simulink model "Single_Cell_BMS"  (R2024a)
settings: Solver=VariableStepAuto  StartTime=0.0  StopTime=1180  RelTol=1e-3
undefined symbols (not defined in the file): C1_LUT, Capacity_LUT, Cell_area, Cell_cp, Cell_mass, DiscIntNeverNeededParam, Em_LUT, H_con, R1_LUT, Ro_LUT, SOC_LUT, T_init, Temp_LUT
settings Model: Creator=gopin  LastModifiedBy=gopin

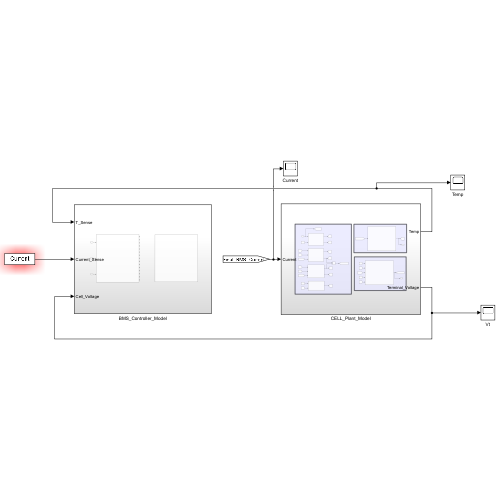
[thumbnail: Simulink's stored preview of the top-level diagram]
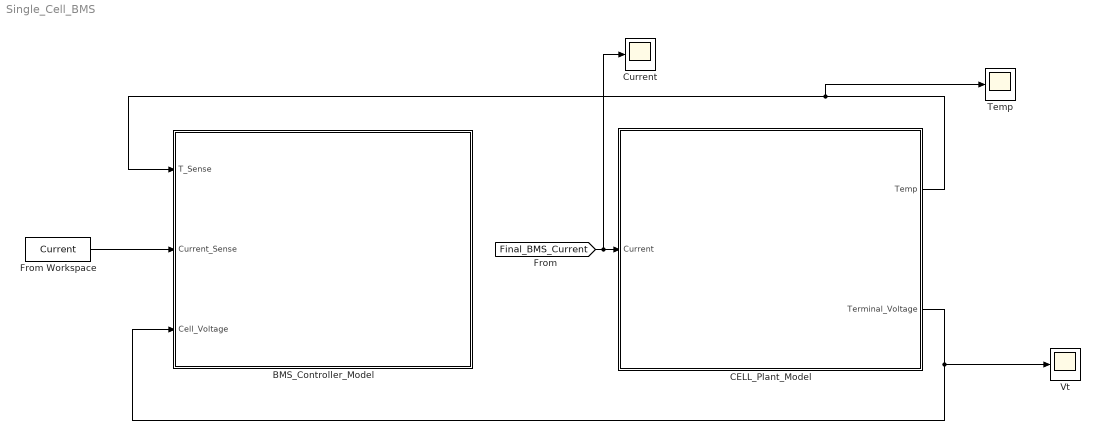
== system Single_Cell_BMS ==
  BMS_Controller_Model : Subsystem
  CELL_Plant_Model : Subsystem
  Current : Scope
  From Workspace : FromWorkspace  VariableName=Current
  Temp : Scope
  Vt : Scope
  wires:
  [Final_BMS_Current] -> Current/1, CELL_Plant_Model/1(Current)
  CELL_Plant_Model/2(Terminal_Voltage) -> BMS_Controller_Model/3(Cell_Voltage), Vt/1
  CELL_Plant_Model/1(Temp) -> Temp/1, BMS_Controller_Model/1(T_Sense)
  From Workspace/1 -> BMS_Controller_Model/2(Current_Sense)

== system Single_Cell_BMS/BMS_Controller_Model ==
  T_Sense : Inport
  Current_Sense : Inport  Port=2
  Cell_Voltage : Inport  Port=3
  Protection_Logc : Subsystem
  SOC_Estimation : Subsystem
  wires:
  Cell_Voltage/1 -> Protection_Logc/1(Cell_voltage)
  Current_Sense/1 -> Protection_Logc/2(C-Sense)
  T_Sense/1 -> Protection_Logc/3(T_Sense)

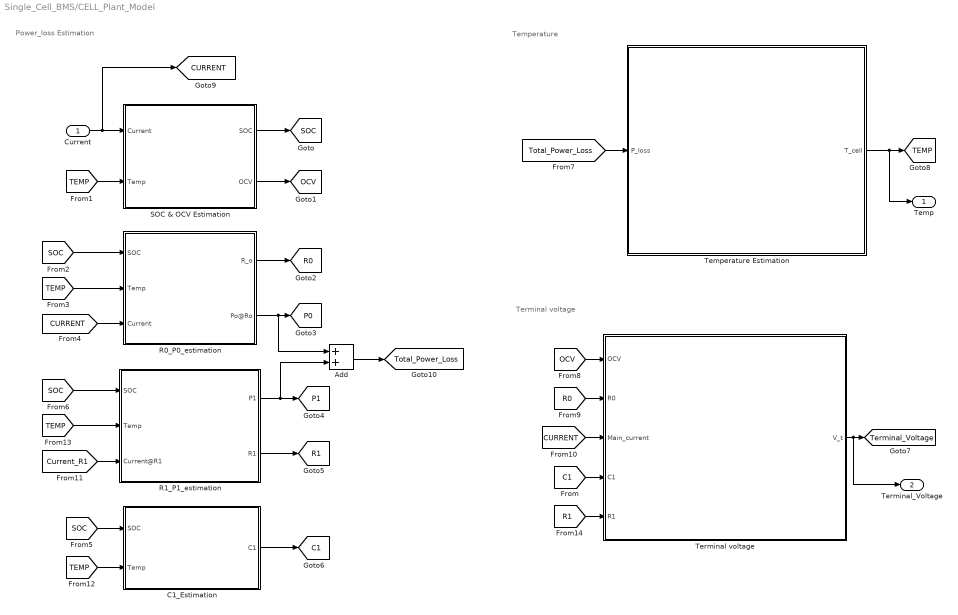
== system Single_Cell_BMS/CELL_Plant_Model ==
  note: Power_loss Estimation
  note: Temperature
  note: Terminal voltage
  Current : Inport
  Add : Sum
  C1_Estimation : Subsystem
  "R0_P0_estimation " : Subsystem
  R1_P1_estimation : Subsystem
  SOC & OCV Estimation : Subsystem
  Temperature Estimation : Subsystem
  Terminal voltage : Subsystem
  Temp : Outport
  Terminal_Voltage : Outport  Port=2
  tag scope: C1=global, CURRENT=global, OCV=global, P0=global, P1=global, R0=global, R1=global, SOC=global, TEMP=global, Terminal_Voltage=global, Total_Power_Loss=global
  wires:
  Current/1 -> [CURRENT], SOC & OCV Estimation/1(Current)
  [TEMP] -> SOC & OCV Estimation/2(Temp)
  [SOC] -> "R0_P0_estimation "/1(SOC)
  [TEMP] -> "R0_P0_estimation "/2(Temp)
  [CURRENT] -> "R0_P0_estimation "/3(Current)
  [SOC] -> R1_P1_estimation/1(SOC)
  [TEMP] -> R1_P1_estimation/2(Temp)
  [Current_R1] -> R1_P1_estimation/3(Current@R1)
  [SOC] -> C1_Estimation/1(SOC)
  [TEMP] -> C1_Estimation/2(Temp)
  [Total_Power_Loss] -> Temperature Estimation/1(P_loss)
  [OCV] -> Terminal voltage/1(OCV)
  [R0] -> Terminal voltage/2(R0)
  [CURRENT] -> Terminal voltage/3(Main_current)
  [C1] -> Terminal voltage/4(C1)
  [R1] -> Terminal voltage/5(R1)
  SOC & OCV Estimation/1(SOC) -> [SOC]
  SOC & OCV Estimation/2(OCV) -> [OCV]
  "R0_P0_estimation "/1(R_o) -> [R0]
  "R0_P0_estimation "/2(Po@Ro) -> Add/1, [P0]
  R1_P1_estimation/1(P1) -> Add/2, [P1]
  R1_P1_estimation/2(R1) -> [R1]
  C1_Estimation/1(C1) -> [C1]
  Temperature Estimation/1(T_cell) -> Temp/1, [TEMP]
  Terminal voltage/1(V_t) -> Terminal_Voltage/1, [Terminal_Voltage]
  Add/1 -> [Total_Power_Loss]

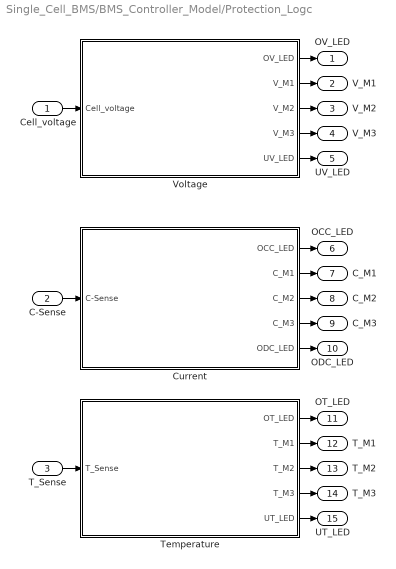
== system Single_Cell_BMS/BMS_Controller_Model/Protection_Logc ==
  Cell_voltage : Inport
  C-Sense : Inport  Port=2
  T_Sense : Inport  Port=3
  Current : Subsystem
  Temperature : Subsystem
  Voltage : Subsystem
  OV_LED : Outport
  V_M1 : Outport  Port=2
  V_M2 : Outport  Port=3
  V_M3 : Outport  Port=4
  UV_LED : Outport  Port=5
  OCC_LED : Outport  Port=6
  C_M1 : Outport  Port=7
  C_M2 : Outport  Port=8
  C_M3 : Outport  Port=9
  ODC_LED : Outport  Port=10
  OT_LED : Outport  Port=11
  T_M1 : Outport  Port=12
  T_M2 : Outport  Port=13
  T_M3 : Outport  Port=14
  UT_LED : Outport  Port=15
  wires:
  Voltage/4(V_M3) -> V_M3/1
  Voltage/1(OV_LED) -> OV_LED/1
  T_Sense/1 -> Temperature/1(T_Sense)
  Voltage/2(V_M1) -> V_M1/1
  Voltage/5(UV_LED) -> UV_LED/1
  Cell_voltage/1 -> Voltage/1(Cell_voltage)
  C-Sense/1 -> Current/1(C-Sense)
  Current/3(C_M2) -> C_M2/1
  Voltage/3(V_M2) -> V_M2/1
  Current/5(ODC_LED) -> ODC_LED/1
  Current/2(C_M1) -> C_M1/1
  Current/4(C_M3) -> C_M3/1
  Temperature/1(OT_LED) -> OT_LED/1
  Temperature/2(T_M1) -> T_M1/1
  Current/1(OCC_LED) -> OCC_LED/1
  Temperature/4(T_M3) -> T_M3/1
  Temperature/3(T_M2) -> T_M2/1
  Temperature/5(UT_LED) -> UT_LED/1

== system Single_Cell_BMS/BMS_Controller_Model/SOC_Estimation ==
  Coloumb Counting Based SOC Estimation : Subsystem
  Voltage Based SOC Estimation : Subsystem

== system Single_Cell_BMS/CELL_Plant_Model/C1_Estimation ==
  SOC : Inport
  Temp : Inport  Port=2
  2-D Lookup Table : Lookup_n-D  BreakpointsForDimension1=SOC_LUT  BreakpointsForDimension2=Temp_LUT  Table=C1_LUT  InternalRulePriority=Speed  RndMeth=Simplest
      settings: InputPortMap=u0,u1
  C1 : Outport
  wires:
  SOC/1 -> 2-D Lookup Table/1
  Temp/1 -> 2-D Lookup Table/2
  2-D Lookup Table/1 -> C1/1

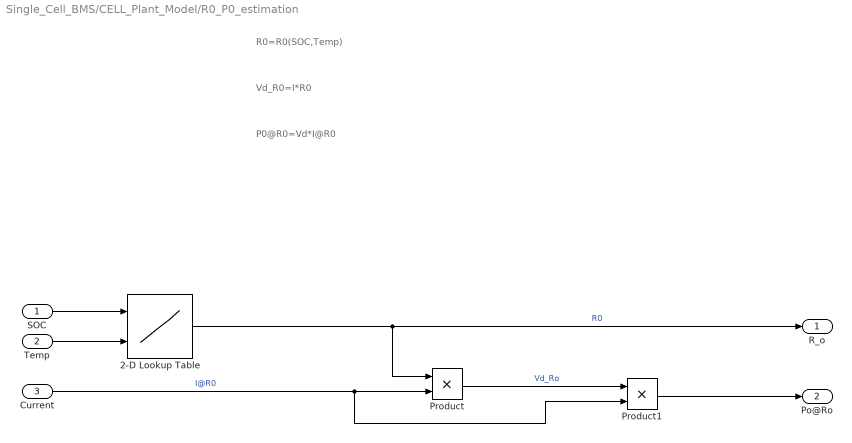
== system Single_Cell_BMS/CELL_Plant_Model/R0_P0_estimation  ==
  note: P0@R0=Vd*I@R0
  note: Vd_R0=I*R0
  note: R0=R0(SOC,Temp)
  SOC : Inport
  Temp : Inport  Port=2
  Current : Inport  Port=3
  2-D Lookup Table : Lookup_n-D  BreakpointsForDimension1=SOC_LUT  BreakpointsForDimension2=Temp_LUT  Table=Ro_LUT  InternalRulePriority=Speed  RndMeth=Simplest
      settings: InputPortMap=u0,u1
  Product : Product
  Product1 : Product
  R_o : Outport
  Po@Ro : Outport  Port=2
  wires:
  Temp/1 -> 2-D Lookup Table/2
  2-D Lookup Table/1 -> Product/1, R_o/1  "R0"
  Current/1 -> Product1/2, Product/2  "I@R0"
  Product/1 -> Product1/1  "Vd_Ro"
  Product1/1 -> Po@Ro/1
  SOC/1 -> 2-D Lookup Table/1

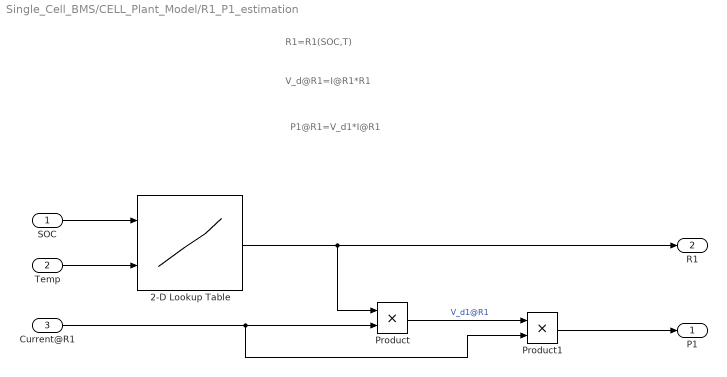
== system Single_Cell_BMS/CELL_Plant_Model/R1_P1_estimation ==
  note: P1@R1=V_d1*I@R1
  note: V_d@R1=I@R1*R1
  note: R1=R1(SOC,T)
  SOC : Inport
  Temp : Inport  Port=2
  Current@R1 : Inport  Port=3
  2-D Lookup Table : Lookup_n-D  BreakpointsForDimension1=SOC_LUT  BreakpointsForDimension2=Temp_LUT  Table=R1_LUT  InternalRulePriority=Speed  RndMeth=Simplest
      settings: InputPortMap=u0,u1
  Product : Product
  Product1 : Product
  P1 : Outport
  R1 : Outport  Port=2
  wires:
  SOC/1 -> 2-D Lookup Table/1
  Temp/1 -> 2-D Lookup Table/2
  2-D Lookup Table/1 -> Product/1, R1/1
  Current@R1/1 -> Product1/2, Product/2
  Product/1 -> Product1/1  "V_d1@R1"
  Product1/1 -> P1/1

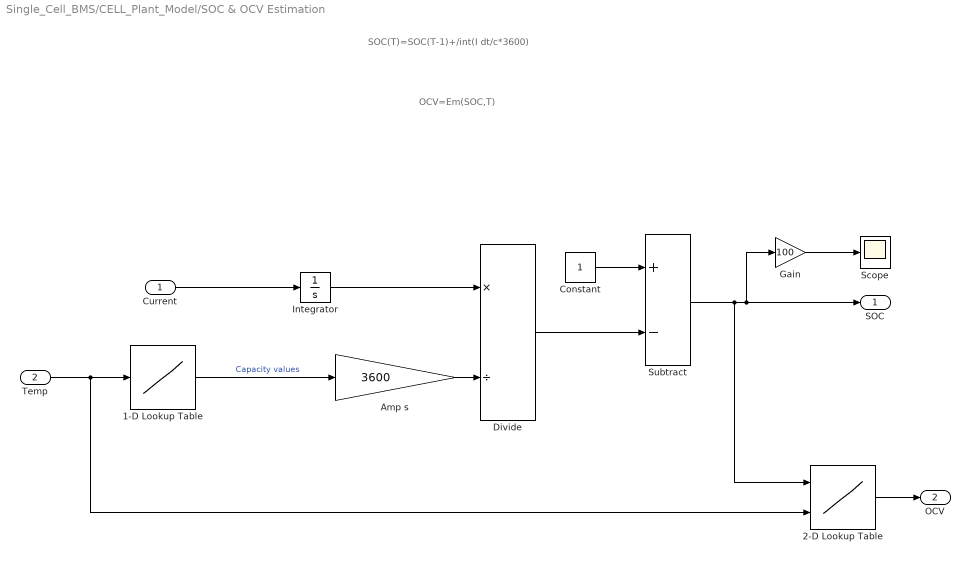
== system Single_Cell_BMS/CELL_Plant_Model/SOC & OCV Estimation ==
  note: SOC(T)=SOC(T-1)+/int(I dt/c*3600)
  note: OCV=Em(SOC,T)
  Current : Inport  OutDataTypeStr=double  PortDimensions=1  SampleTime=0
  Temp : Inport  Port=2  OutDataTypeStr=double  PortDimensions=1  SampleTime=0
  1-D Lookup Table : Lookup_n-D  NumberOfTableDimensions=1  BreakpointsForDimension1=Temp_LUT  Table=Capacity_LUT  InternalRulePriority=Speed  RndMeth=Simplest
  2-D Lookup Table : Lookup_n-D  BreakpointsForDimension1=SOC_LUT  BreakpointsForDimension2=Temp_LUT  Table=Em_LUT  InternalRulePriority=Speed  RndMeth=Simplest
      settings: InputPortMap=u0,u1
  Amp s : Gain  Gain=3600
  Constant : Constant
  Divide : Product  Inputs=*/
  Gain : Gain  Gain=100
  Integrator : Integrator
  Scope : Scope
  Subtract : Sum  Inputs=+-
  SOC : Outport  OutDataTypeStr=double  PortDimensions=1  SampleTime=0
  OCV : Outport  Port=2  OutDataTypeStr=double  PortDimensions=1  SampleTime=0
  wires:
  2-D Lookup Table/1 -> OCV/1
  1-D Lookup Table/1 -> Amp s/1  "Capacity values"
  Subtract/1 -> Gain/1, SOC/1, 2-D Lookup Table/1
  Gain/1 -> Scope/1
  Current/1 -> Integrator/1
  Amp s/1 -> Divide/2
  Temp/1 -> 1-D Lookup Table/1, 2-D Lookup Table/2
  Integrator/1 -> Divide/1
  Divide/1 -> Subtract/2
  Constant/1 -> Subtract/1

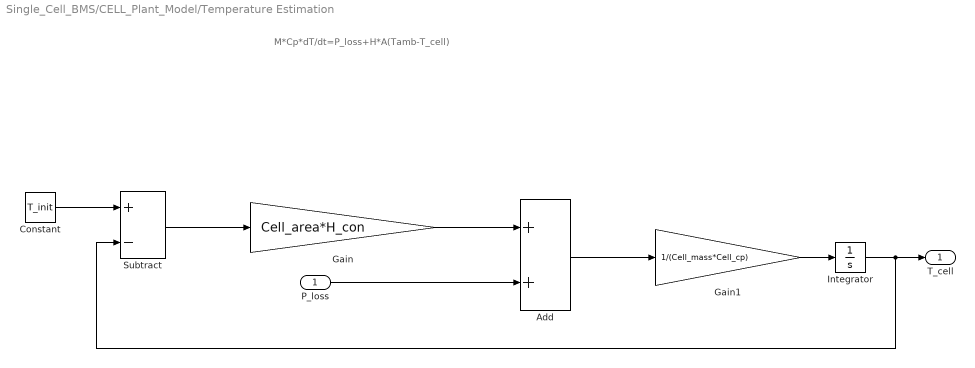
== system Single_Cell_BMS/CELL_Plant_Model/Temperature Estimation ==
  note: M*Cp*dT/dt=P_loss+H*A(Tamb-T_cell)
  P_loss : Inport  OutDataTypeStr=double  PortDimensions=1  SampleTime=0
  Add : Sum
  Constant : Constant  Value=T_init
  Gain : Gain  Gain=Cell_area*H_con
  Gain1 : Gain  Gain=1/(Cell_mass*Cell_cp)
  Integrator : Integrator  InitialCondition=293.15
  Subtract : Sum  Inputs=+-
  T_cell : Outport  OutDataTypeStr=double  PortDimensions=1  SampleTime=0
  wires:
  P_loss/1 -> Add/2
  Add/1 -> Gain1/1
  Integrator/1 -> T_cell/1, Subtract/2
  Gain1/1 -> Integrator/1
  Subtract/1 -> Gain/1
  Gain/1 -> Add/1
  Constant/1 -> Subtract/1

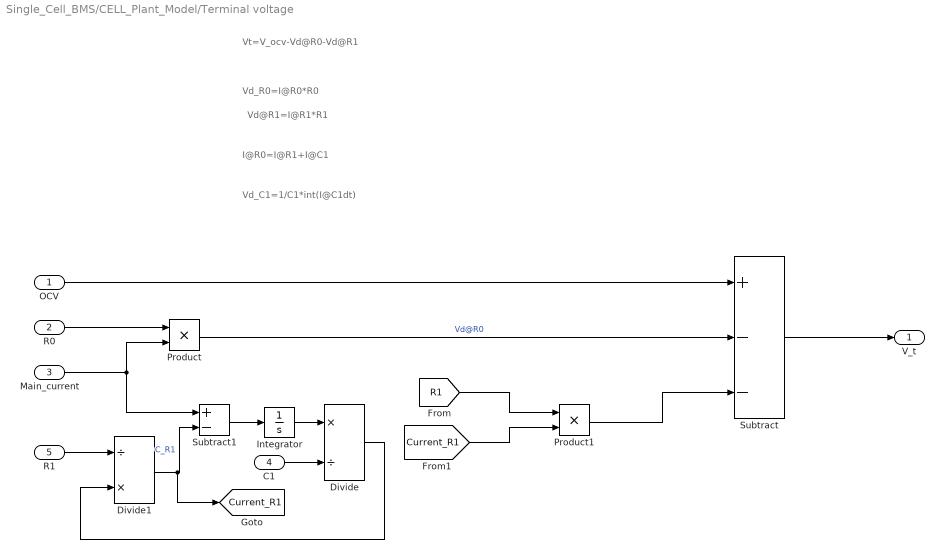
== system Single_Cell_BMS/CELL_Plant_Model/Terminal voltage ==
  note: Vd_C1=1/C1*int(I@C1dt)
  note: I@R0=I@R1+I@C1
  note: Vd@R1=I@R1*R1
  note: Vd_R0=I@R0*R0
  note: Vt=V_ocv-Vd@R0-Vd@R1
  OCV : Inport
  R0 : Inport  Port=2
  Main_current : Inport  Port=3
  C1 : Inport  Port=4
  R1 : Inport  Port=5
  Divide : Product  Inputs=*/
  Divide1 : Product  Inputs=/*
  Integrator : Integrator
  Product : Product
  Product1 : Product
  Subtract : Sum  Inputs=+--
  Subtract1 : Sum  Inputs=+-
  V_t : Outport
  tag scope: Current_R1=global
  wires:
  Subtract/1 -> V_t/1
  OCV/1 -> Subtract/1
  R0/1 -> Product/1
  Main_current/1 -> Subtract1/1, Product/2
  Product/1 -> Subtract/2  "Vd@R0"
  [R1] -> Product1/1
  [Current_R1] -> Product1/2
  Product1/1 -> Subtract/3
  Subtract1/1 -> Integrator/1
  Integrator/1 -> Divide/1
  C1/1 -> Divide/2
  Divide1/1 -> [Current_R1], Subtract1/2  "C_R1"
  R1/1 -> Divide1/1
  Divide/1 -> Divide1/2

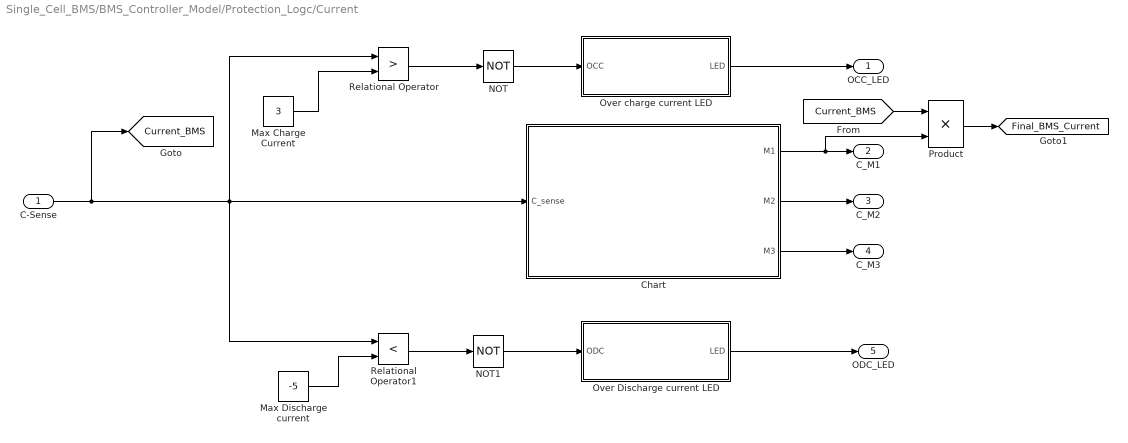
== system Single_Cell_BMS/BMS_Controller_Model/Protection_Logc/Current ==
  C-Sense : Inport
  Chart : Stateflow chart  TreatAsAtomicUnit=on
  Max Charge Current : Constant  Value=3
  Max Discharge current : Constant  Value=-5
  NOT : Logic  Operator=NOT  AllPortsSameDT=off  OutDataTypeStr=boolean
  NOT1 : Logic  Operator=NOT  AllPortsSameDT=off  OutDataTypeStr=boolean
  Over Discharge current LED : Stateflow chart  TreatAsAtomicUnit=on
  Over charge current LED : Stateflow chart  TreatAsAtomicUnit=on
  Product : Product
  Relational Operator : RelationalOperator  Operator=>  OutDataTypeStr=boolean  RndMeth=Simplest  InputSameDT=off
  Relational Operator1 : RelationalOperator  Operator=<  OutDataTypeStr=boolean  RndMeth=Simplest  InputSameDT=off
  OCC_LED : Outport
  C_M1 : Outport  Port=2
  C_M2 : Outport  Port=3
  C_M3 : Outport  Port=4
  ODC_LED : Outport  Port=5
  tag scope: Current_BMS=global, Final_BMS_Current=global
  wires:
  Over charge current LED/1(LED) -> OCC_LED/1
  Relational Operator1/1 -> NOT1/1
  Relational Operator/1 -> NOT/1
  Chart/1(M1) -> Product/2, C_M1/1
  Max Discharge current/1 -> Relational Operator1/2
  Chart/2(M2) -> C_M2/1
  Chart/3(M3) -> C_M3/1
  C-Sense/1 -> [Current_BMS], Chart/1(C_sense), Relational Operator1/1, Relational Operator/1
  Over Discharge current LED/1(LED) -> ODC_LED/1
  Max Charge Current/1 -> Relational Operator/2
  [Current_BMS] -> Product/1
  Product/1 -> [Final_BMS_Current]
  NOT/1 -> Over charge current LED/1(OCC)
  NOT1/1 -> Over Discharge current LED/1(ODC)

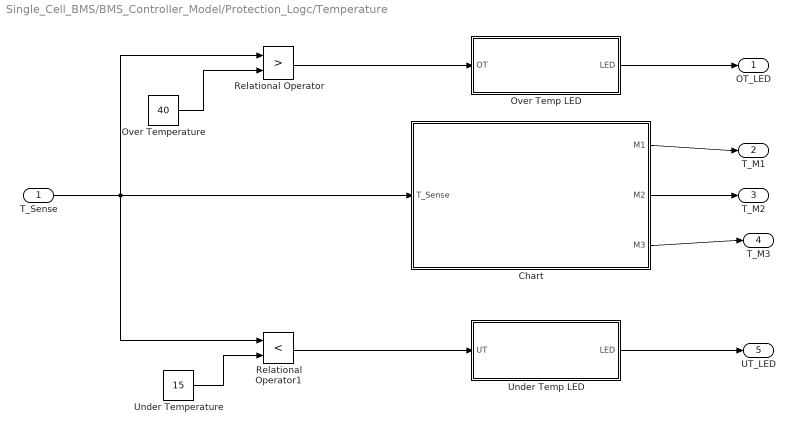
== system Single_Cell_BMS/BMS_Controller_Model/Protection_Logc/Temperature ==
  T_Sense : Inport
  Chart : Stateflow chart  TreatAsAtomicUnit=on
  Over Temp LED : Stateflow chart  TreatAsAtomicUnit=on
  Over Temperature : Constant  Value=40
  Relational Operator : RelationalOperator  Operator=>  OutDataTypeStr=boolean  RndMeth=Simplest  InputSameDT=off
  Relational Operator1 : RelationalOperator  Operator=<  OutDataTypeStr=boolean  RndMeth=Simplest  InputSameDT=off
  Under Temp LED : Stateflow chart  TreatAsAtomicUnit=on
  Under Temperature : Constant  Value=15
  OT_LED : Outport
  T_M1 : Outport  Port=2
  T_M2 : Outport  Port=3
  T_M3 : Outport  Port=4
  UT_LED : Outport  Port=5
  wires:
  Over Temp LED/1(LED) -> OT_LED/1
  Relational Operator1/1 -> Under Temp LED/1(UT)
  Relational Operator/1 -> Over Temp LED/1(OT)
  Chart/1(M1) -> T_M1/1
  Under Temperature/1 -> Relational Operator1/2
  Chart/2(M2) -> T_M2/1
  Chart/3(M3) -> T_M3/1
  T_Sense/1 -> Relational Operator1/1, Chart/1(T_Sense), Relational Operator/1
  Under Temp LED/1(LED) -> UT_LED/1
  Over Temperature/1 -> Relational Operator/2

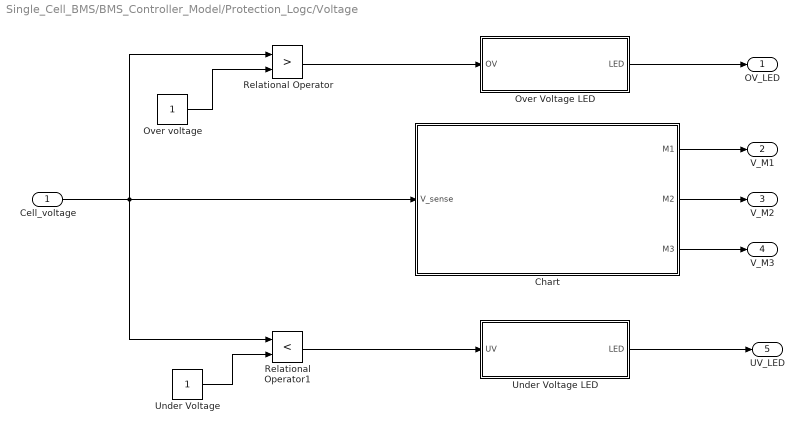
== system Single_Cell_BMS/BMS_Controller_Model/Protection_Logc/Voltage ==
  Cell_voltage : Inport
  Chart : Stateflow chart  TreatAsAtomicUnit=on
  Over Voltage LED : Stateflow chart  TreatAsAtomicUnit=on
  Over voltage : Constant
  Relational Operator : RelationalOperator  Operator=>  OutDataTypeStr=boolean  RndMeth=Simplest  InputSameDT=off
  Relational Operator1 : RelationalOperator  Operator=<  OutDataTypeStr=boolean  RndMeth=Simplest  InputSameDT=off
  Under Voltage : Constant
  Under Voltage LED : Stateflow chart  TreatAsAtomicUnit=on
  OV_LED : Outport
  V_M1 : Outport  Port=2
  V_M2 : Outport  Port=3
  V_M3 : Outport  Port=4
  UV_LED : Outport  Port=5
  wires:
  Cell_voltage/1 -> Relational Operator/1, Relational Operator1/1, Chart/1(V_sense)
  Under Voltage/1 -> Relational Operator1/2
  Over voltage/1 -> Relational Operator/2
  Relational Operator/1 -> Over Voltage LED/1(OV)
  Relational Operator1/1 -> Under Voltage LED/1(UV)
  Over Voltage LED/1(LED) -> OV_LED/1
  Chart/1(M1) -> V_M1/1
  Chart/2(M2) -> V_M2/1
  Chart/3(M3) -> V_M3/1
  Under Voltage LED/1(LED) -> UV_LED/1

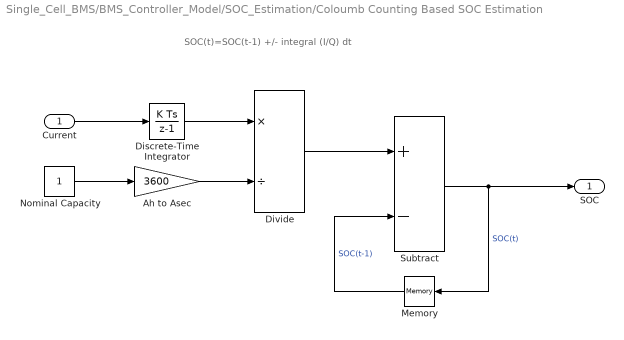
== system Single_Cell_BMS/BMS_Controller_Model/SOC_Estimation/Coloumb Counting Based SOC Estimation ==
  note: SOC(t)=SOC(t-1) +/- integral (I/Q) dt
  Current : Inport
  Ah to Asec : Gain  Gain=3600
  Discrete-Time Integrator : DiscreteIntegrator  SampleTime=-1  ICPrevOutput=DiscIntNeverNeededParam  ICPrevScaledInput=DiscIntNeverNeededParam
  Divide : Product  Inputs=*/
  Memory : Memory
  Nominal Capacity : Constant
  Subtract : Sum  Inputs=+-
  SOC : Outport
  wires:
  Current/1 -> Discrete-Time Integrator/1
  Discrete-Time Integrator/1 -> Divide/1
  Ah to Asec/1 -> Divide/2
  Nominal Capacity/1 -> Ah to Asec/1
  Divide/1 -> Subtract/1
  Subtract/1 -> Memory/1, SOC/1  "SOC(t)"
  Memory/1 -> Subtract/2  "SOC(t-1)"

== system Single_Cell_BMS/BMS_Controller_Model/SOC_Estimation/Voltage Based SOC Estimation ==
  note: SOC(Fn(Voltage))
  1-D Lookup Table : Lookup_n-D  NumberOfTableDimensions=1  BreakpointsForDimension1=[-5:5]  Table=tanh([-5:5])  InternalRulePriority=Speed  RndMeth=Simplest
  Display : Display
  Voltage Sense : From
  SOC : Outport
  wires:
  1-D Lookup Table/1 -> SOC/1, Display/1  "SOC in %"
  Voltage Sense/1 -> 1-D Lookup Table/1  "Voltage Data"

== stateflow chart Single_Cell_BMS/BMS_Controller_Model/Protection_Logc/Voltage/Under Voltage LED ==
  state LED_OFF
    en:
    LED=0;
    du:
    LED=0;
  state LED_ON
    en:
    LED=1;
  (default) -> LED_OFF
  LED_OFF -> LED_ON : [UV==1]
  LED_ON -> LED_OFF : [UV==0]
  data: LED output; UV input

== stateflow chart Single_Cell_BMS/BMS_Controller_Model/Protection_Logc/Current/Over charge current LED ==
  state LED_OFF
    en:
    LED=0;
    du:
    LED=0;
  state LED_ON
    en:
    LED=1;
  (default) -> LED_OFF
  LED_OFF -> LED_ON : [OCC==1]
  LED_ON -> LED_OFF : [OCC==0]
  data: LED output; OCC input

== stateflow chart Single_Cell_BMS/BMS_Controller_Model/Protection_Logc/Current/Over Discharge current LED ==
  state LED_OFF
    en:
    LED=0;
    du:
    LED=0;
  state LED_ON
    en:
    LED=1;
  (default) -> LED_OFF
  LED_OFF -> LED_ON : [ODC==1]
  LED_ON -> LED_OFF : [ODC==0]
  data: LED output; ODC input

== stateflow chart Single_Cell_BMS/BMS_Controller_Model/Protection_Logc/Temperature/Over Temp LED ==
  state LED_OFF
    en:
    LED=0;
    du:
    LED=0;
  state LED_ON
    en:
    LED=1;
  (default) -> LED_OFF
  LED_OFF -> LED_ON : [OT==1]
  LED_ON -> LED_OFF : [OT==0]
  data: LED output; OT input

== stateflow chart Single_Cell_BMS/BMS_Controller_Model/Protection_Logc/Temperature/Under Temp LED ==
  state LED_OFF
    en:
    LED=0;
    du:
    LED=0;
  state LED_ON
    en:
    LED=1;
  (default) -> LED_OFF
  LED_OFF -> LED_ON : [UT==1]
  LED_ON -> LED_OFF : [UT==0]
  data: LED output; UT input

== stateflow chart Single_Cell_BMS/BMS_Controller_Model/Protection_Logc/Current/Chart ==
  state Charge_Only
    en:
    M1=1;
    M2=1;
    M3=0;
  state Charge_cutoff
    en:
    M1=0;
    M2=0;
  state Initial_Start
    en:
    M1=1;
    M2=1;
    M3=1;
  state Discharge_Only
    en:
    M1=1;
    M2=0;
    M3=1;
  state Discharge_cutoff
    en:
    M1=0;
    M3=0;
  Initial_Start -> Charge_Only [order 1] : [C_sense<2.5&&C_sense>0.5]
  Charge_Only -> Charge_cutoff [order 2] : [C_sense>2.5]
  Charge_cutoff -> Charge_Only [order 1] : [C_sense<2.5&&C_sense>0.5&&after(10,sec)]
  Charge_Only -> Initial_Start [order 3] : [C_sense<0.5]
  (default) -> Initial_Start
  Charge_cutoff -> Discharge_Only [order 2] : [C_sense>-5&&C_sense<-0.5]
  Charge_Only -> Discharge_Only [order 1] : [C_sense<2.5&&C_sense>0.5]
  Discharge_Only -> Charge_Only [order 2] : [C_sense>-5&&C_sense<-0.5]
  Discharge_cutoff -> Charge_Only [order 2] : [C_sense<2.5&&C_sense>0.5]
  Initial_Start -> Discharge_Only [order 2] : [C_sense>-5&&C_sense<-0.2]
  Discharge_Only -> Initial_Start [order 1] : [C_sense>-0.2]
  Discharge_Only -> Discharge_cutoff [order 3] : [C_sense<-5]
  Discharge_cutoff -> Discharge_Only [order 1] : [C_sense>-5&&C_sense<-0.2&&after(10,sec)]
  data: C_sense input; M1 output; M2 output; M3 output

== stateflow chart Single_Cell_BMS/BMS_Controller_Model/Protection_Logc/Temperature/Chart ==
  state OT_Cutoff
    en:
    M1=0;
    M2=0;
    M3=0;
  state Initial_Start
    en:
    M1=1;
    M2=1;
    M3=1;
  state UT_Cutoff
    en:
    M1=0;
    M2=0;
    M3=0;
  Initial_Start -> OT_Cutoff [order 1] : [T_Sense>40]
  (default) -> Initial_Start
  OT_Cutoff -> Initial_Start : [T_Sense<35&&after(10,sec)]
  UT_Cutoff -> Initial_Start : [T_Sense>15&&after(10,sec)]
  Initial_Start -> UT_Cutoff [order 2] : [T_Sense<15]
  data: T_Sense input; M1 output; M2 output; M3 output

== stateflow chart Single_Cell_BMS/BMS_Controller_Model/Protection_Logc/Voltage/Chart ==
  state Charge_Cutoff
    en:
    M1=0;
    M2=0;
    M3=1;
  state Initial_Start
    en:
    M1=1;
    M2=1;
    M3=1;
  state Only_discharge
    en:
    M1=1;
    M3=1;
  state Discharge_Cutoff
    en:
    M1=0;
    M2=1;
    M3=0;
  state Only_discharge1
    en:
    M1=1;
    M3=1;
  Initial_Start -> Charge_Cutoff [order 1] : [V_sense>4.15]
  (default) -> Initial_Start
  Charge_Cutoff -> Initial_Start [order 1] : [V_sense<4.0&&after(10,sec)]
  Only_discharge -> Initial_Start : [V_sense<4&&V_sense>3]
  Charge_Cutoff -> Only_discharge [order 2] : [after(15,sec)&&V_sense<=4.1]
  Only_discharge1 -> Initial_Start : [V_sense<4&&V_sense>3]
  Discharge_Cutoff -> Only_discharge1 [order 2] : [after(15,sec)&&V_sense>=2.85]
  Initial_Start -> Discharge_Cutoff [order 2] : [V_sense>2.8]
  Discharge_Cutoff -> Initial_Start [order 1] : [V_sense>3.0&&after(10,sec)]
  data: M1 output; V_sense input; M2 output; M3 output

== stateflow chart Single_Cell_BMS/BMS_Controller_Model/Protection_Logc/Voltage/Over Voltage LED ==
  state LED_OFF
    en:
    LED=0;
    du:
    LED=0;
  state LED_ON
    en:
    LED=1;
  (default) -> LED_OFF
  LED_OFF -> LED_ON : [OV==1]
  LED_ON -> LED_OFF : [OV==0]
  data: LED output; OV input
